simulink model "DP_sim"  (R2020b)
settings: Solver=VariableStepAuto  StartTime=0.0  StopTime=10.0  RelTol=1e-5
values from neighbouring files (symbols this model uses):
  d_theta1_0 = -2    [DoublePendulum.m]
  d_theta2_0 = -1    [DoublePendulum.m]
  theta1_0 = theta1_0 +phi    (= 1.67079632679)    [DoublePendulum.m]
  theta2_0 = theta2_0 +phi    (= 1.67079632679)    [DoublePendulum.m]
settings Model: Creator=valen  LastModifiedBy=valen

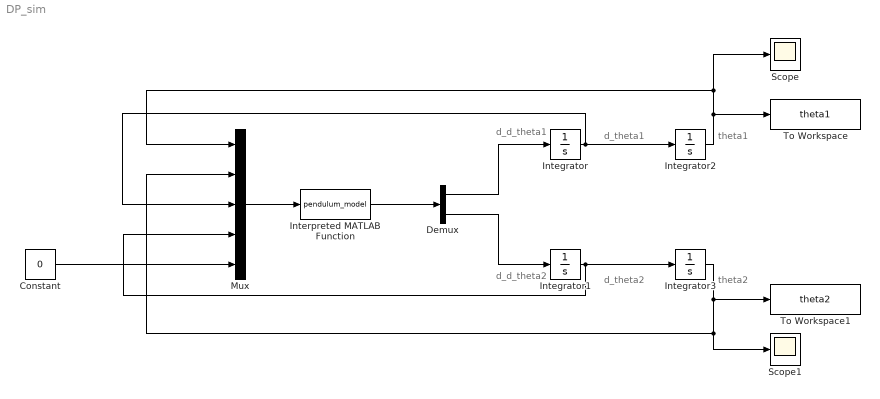
== system DP_sim ==
  note: d_d_theta2
  note: d_d_theta1
  note: d_theta2
  note: d_theta1
  note: theta2
  note: theta1
  Constant : Constant  Value=0
  Demux : Demux  Outputs=2
  Integrator : Integrator  InitialCondition=d_theta1_0
  Integrator1 : Integrator  InitialCondition=d_theta2_0
  Integrator2 : Integrator  InitialCondition=theta1_0
  Integrator3 : Integrator  InitialCondition=theta2_0
  Interpreted MATLAB Function : MATLABFcn  MATLABFcn=pendulum_model
  Mux : Mux  Inputs=5
  Scope : Scope
  Scope1 : Scope
  To Workspace : ToWorkspace  VariableName=theta1  SaveFormat=Structure With Time  SampleTime=-1
  To Workspace1 : ToWorkspace  VariableName=theta2  SaveFormat=Structure With Time  SampleTime=-1
  wires:
  Interpreted MATLAB Function/1 -> Demux/1
  Demux/1 -> Integrator/1
  Integrator/1 -> Mux/3, Integrator2/1
  Demux/2 -> Integrator1/1
  Integrator1/1 -> Mux/4, Integrator3/1
  Integrator2/1 -> Scope/1, Mux/1, To Workspace/1
  Integrator3/1 -> Scope1/1, Mux/2, To Workspace1/1
  Constant/1 -> Mux/5
  Mux/1 -> Interpreted MATLAB Function/1
